simulink model "RealtimeModel"  (Simulink 7.0)
settings: Solver=FixedStepDiscrete  SolverMode=MultiTasking  StartTime=0.0  StopTime=RunningTime  FixedStep=sample  RelTol=1e-3
values from neighbouring files (symbols this model uses):
  Integrator = InitializeIntegrator(Integrator, Structure)    [RealtimeModel_Setup.m]
  SampleRate = Integrator.Timestep    [RealtimeModel_Setup.m]
  Structure = CalculateMatrices(Structure, Elements)    [RealtimeModel_Setup.m]
undefined symbols (not defined in the file or in its folder): Elements
libraries: simulink x2
(part 1 of 11)
settings Model: Creator=Tommy  LastModifiedBy=Tommy  BufferReuse=off
settings OptimizationCC: BlockReduction=off  OptimizeBlockIOStorage=off  BufferReuse=off  ExpressionFolding=off  LocalBlockOutputs=off
settings RTWCC: SystemTargetFile=xpctarget.tlc  TemplateMakefile=xpc_default_tmf  Description=xPC Target  ProcessScript=xpctarget_make_rtw_hook
settings xpcTargetCC: TargetFcnLib=ansi_tfl_table_tmw.mat  GenFloatMathFcnCalls=ANSI_C  CompOptLevelCompliant=off  PortableWordSizes=off
settings CustomProperty: DataType=string  Value=Real-Time

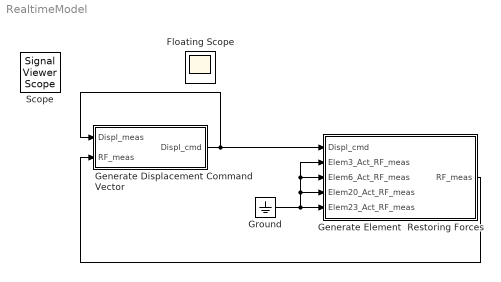
== system RealtimeModel ==
  Generate Displacement Command Vector : Subsystem
      mask Type: Generate Displacement Command Vector
      mask Description:
      | Generates the Displacement vector using the CR Algorithm.
      | 
      | Connect the measured displacement vector and measured restoring force vector to the inputs.
  Generate Element  Restoring Forces : Subsystem  TreatAsAtomicUnit=on  SystemSampleTime=SampleRate
  Ground : Ground
  Floating Scope : Scope
      settings: Floating=on
  Scope : SignalViewerScope  IOType=viewer  SampleTime=-1  RefreshTime=0.035000
  wires:
  Generate Displacement Command Vector/1(Displ_cmd) -> Generate Displacement Command Vector/1(Displ_meas), Generate Element  Restoring Forces/1(Displ_cmd)
  Generate Element  Restoring Forces/1(RF_meas) -> Generate Displacement Command Vector/2(RF_meas)
  Ground/1 -> Generate Element  Restoring Forces/5(Elem23_Act_RF_meas), Generate Element  Restoring Forces/4(Elem20_Act_RF_meas), Generate Element  Restoring Forces/3(Elem6_Act_RF_meas), Generate Element  Restoring Forces/2(Elem3_Act_RF_meas)

== system RealtimeModel/Generate Displacement Command Vector ==
  Displ_meas : Inport  OutDataType=sfix(16)  OutScaling=2^0
  RF_meas : Inport  Port=2  OutDataType=sfix(16)  OutScaling=2^0
  Constant : Constant  Value=Integrator.Alpha1  OutDataType=sfix(16)  OutScaling=2^0
  Constant1 : Constant  Value=Integrator.Alpha2  OutDataType=sfix(16)  OutScaling=2^0
  Constant2 : Constant  Value=Integrator.Timestep  OutDataType=sfix(16)  OutScaling=2^0
  Constant3 : Constant  Value=Integrator.PEFF  OutDataType=sfix(16)  OutScaling=2^0
  Data Store Acceleration : DataStoreMemory  DataStoreName=Acceleration  InitialValue=Integrator.Acceleration  OutDataType=sfix(16)  OutScaling=2^0
  Data Store DampingMatrixFree : DataStoreMemory  DataStoreName=DampingMatrixFree  InitialValue=Structure.DampingMatrixFree  OutDataType=sfix(16)  OutScaling=2^0
  Data Store Displacement : DataStoreMemory  DataStoreName=Displacement  InitialValue=Integrator.Displacement  OutDataType=sfix(16)  OutScaling=2^0
  Data Store MassMatrixFreeInv : DataStoreMemory  DataStoreName=MassMatrixFreeInv  InitialValue=Structure.MassMatrixFreeInv  OutDataType=sfix(16)  OutScaling=2^0
  Data Store Read Acceleration : DataStoreRead  DataStoreName=Acceleration  SampleTime=SampleRate
  Data Store Read DampingMatrixFree : DataStoreRead  DataStoreName=DampingMatrixFree  SampleTime=SampleRate
  Data Store Read Displacement : DataStoreRead  DataStoreName=Displacement  SampleTime=SampleRate
  Data Store Read MassMatrixFreeInv : DataStoreRead  DataStoreName=MassMatrixFreeInv  SampleTime=SampleRate
  Data Store Read Velocity : DataStoreRead  DataStoreName=Velocity  SampleTime=SampleRate
  Data Store Velocity : DataStoreMemory  DataStoreName=Velocity  InitialValue=Integrator.Velocity  OutDataType=sfix(16)  OutScaling=2^0
  Data Store Write Acceleration : DataStoreWrite  DataStoreName=Acceleration  SampleTime=-1
  Data Store Write Displacement : DataStoreWrite  DataStoreName=Displacement  SampleTime=-1
  Data Store Write Velocity : DataStoreWrite  DataStoreName=Velocity  SampleTime=-1
  Generate Acceleration Vector : Stateflow chart  TreatAsAtomicUnit=on  SystemSampleTime=SampleRate
  Generate Command Vectors : Stateflow chart  TreatAsAtomicUnit=on  SystemSampleTime=SampleRate
  Integration Step Count : Subsystem  TreatAsAtomicUnit=on  SystemSampleTime=SampleRate
      mask Type: Step count
      mask Description: Generates the step count
  Displ_cmd : Outport  OutDataType=sfix(16)  OutScaling=2^0
  wires:
  Generate Command Vectors/1(Displacement_v) -> Displ_cmd/1
  Constant2/1 -> Generate Command Vectors/1(Timestep)
  Constant1/1 -> Generate Command Vectors/3(Alpha2)
  Data Store Read Displacement/1 -> Generate Command Vectors/4(Displacement)
  Data Store Read Velocity/1 -> Generate Command Vectors/5(Velocity)
  Data Store Read Acceleration/1 -> Generate Command Vectors/6(Acceleration)
  Constant/1 -> Generate Command Vectors/2(Alpha1)
  Displ_meas/1 -> Data Store Write Displacement/1
  RF_meas/1 -> Generate Acceleration Vector/2(TotalRF)
  Generate Command Vectors/2(Velocity_v) -> Data Store Write Velocity/1, Generate Acceleration Vector/1(Velocity)
  Generate Acceleration Vector/1(Acceleration) -> Data Store Write Acceleration/1
  Constant3/1 -> Generate Acceleration Vector/3(PEFF)
  Data Store Read MassMatrixFreeInv/1 -> Generate Acceleration Vector/4(M_FreeInv)
  Data Store Read DampingMatrixFree/1 -> Generate Acceleration Vector/5(C_Free)
  Integration Step Count/1(Step Count) -> Generate Acceleration Vector/6(step_count)

== system RealtimeModel/Generate Element  Restoring Forces ==
  Displ_cmd : Inport  OutDataType=sfix(16)  OutScaling=2^0
  Elem3_Act_RF_meas : Inport  Port=2  OutDataType=sfix(16)  OutScaling=2^0
  Elem6_Act_RF_meas : Inport  Port=3  OutDataType=sfix(16)  OutScaling=2^0
  Elem20_Act_RF_meas : Inport  Port=4  OutDataType=sfix(16)  OutScaling=2^0
  Elem23_Act_RF_meas : Inport  Port=5  OutDataType=sfix(16)  OutScaling=2^0
  Form Total Restoring Force Vector : Subsystem  TreatAsAtomicUnit=on  SystemSampleTime=SampleRate
      mask Type: Form Restoring Force Vector
      mask Description:
      | Takes the restoring force vectors from each Element and combines them to form a total restoring force vector.
      | 
      | Connect the "Nodes_muxed" signal to the output of a Mux block which takes in all the Element "Nodes" outputs in order of ID.
      | 
      | Connect the "RF_muxed" signal to the output of a Mux block which takes in all the Element "RF" outputs in order of ID.
  Generate Type 1  Element Restoring Force Element 11 : Subsystem  TreatAsAtomicUnit=on  SystemSampleTime=SampleRate  mask(Generate Type 1 Element Restoring Force){id=11}
      mask prompts: id "Element ID"
      mask help:
      | Generates the Restoring Force vector for a Type 1 Element
      |
      | Enter the ID for this element corresponding with the input configuration file
  Generate Type 1  Element Restoring Force Element 12 : Subsystem  TreatAsAtomicUnit=on  SystemSampleTime=SampleRate  mask(Generate Type 1 Element Restoring Force){id=12}
      mask prompts: id "Element ID"
      mask help:
      | Generates the Restoring Force vector for a Type 1 Element
      |
      | Enter the ID for this element corresponding with the input configuration file
  Generate Type 1  Element Restoring Force Element 14 : Subsystem  TreatAsAtomicUnit=on  SystemSampleTime=SampleRate  mask(Generate Type 1 Element Restoring Force){id=14}
      mask prompts: id "Element ID"
      mask help:
      | Generates the Restoring Force vector for a Type 1 Element
      |
      | Enter the ID for this element corresponding with the input configuration file
  Generate Type 1  Element Restoring Force Element 15 : Subsystem  TreatAsAtomicUnit=on  SystemSampleTime=SampleRate  mask(Generate Type 1 Element Restoring Force){id=15}
      mask prompts: id "Element ID"
      mask help:
      | Generates the Restoring Force vector for a Type 1 Element
      |
      | Enter the ID for this element corresponding with the input configuration file
  Generate Type 1  Element Restoring Force Element 28 : Subsystem  TreatAsAtomicUnit=on  SystemSampleTime=SampleRate  mask(Generate Type 1 Element Restoring Force){id=28}
      mask prompts: id "Element ID"
      mask help:
      | Generates the Restoring Force vector for a Type 1 Element
      |
      | Enter the ID for this element corresponding with the input configuration file
  Generate Type 1  Element Restoring Force Element 29 : Subsystem  TreatAsAtomicUnit=on  SystemSampleTime=SampleRate  mask(Generate Type 1 Element Restoring Force){id=29}
      mask prompts: id "Element ID"
      mask help:
      | Generates the Restoring Force vector for a Type 1 Element
      |
      | Enter the ID for this element corresponding with the input configuration file
  Generate Type 1  Element Restoring Force Element 31 : Subsystem  TreatAsAtomicUnit=on  SystemSampleTime=SampleRate  mask(Generate Type 1 Element Restoring Force){id=31}
      mask prompts: id "Element ID"
      mask help:
      | Generates the Restoring Force vector for a Type 1 Element
      |
      | Enter the ID for this element corresponding with the input configuration file
  Generate Type 1  Element Restoring Force Element 32 : Subsystem  TreatAsAtomicUnit=on  SystemSampleTime=SampleRate  mask(Generate Type 1 Element Restoring Force){id=32}
      mask prompts: id "Element ID"
      mask help:
      | Generates the Restoring Force vector for a Type 1 Element
      |
      | Enter the ID for this element corresponding with the input configuration file
  Generate Type 2 Element Restoring Force Element 20 : Subsystem  TreatAsAtomicUnit=on  SystemSampleTime=SampleRate  mask(Generate Type 2 Element Restoring Force){id=20, simulation=off}
      mask prompts: id "Element ID"; simulation "Experiment Mode"
      mask help:
      | Generates the Restoring Force vector for a Type 2 Element
      |
      | Enter the ID for this element corresponding with the input configuration file
      |
      | Check the "Experiment Mode" box to activate the Act_RF_meas input.
      | Connect the Actuator Restoring Force feedback to the input.
  Generate Type 2 Element Restoring Force Element 23 : Subsystem  TreatAsAtomicUnit=on  SystemSampleTime=SampleRate  mask(Generate Type 2 Element Restoring Force){id=23, simulation=off}
      mask prompts: id "Element ID"; simulation "Experiment Mode"
      mask help:
      | Generates the Restoring Force vector for a Type 2 Element
      |
      | Enter the ID for this element corresponding with the input configuration file
      |
      | Check the "Experiment Mode" box to activate the Act_RF_meas input.
      | Connect the Actuator Restoring Force feedback to the input.
  Generate Type 2 Element Restoring Force Element 3 : Subsystem  TreatAsAtomicUnit=on  SystemSampleTime=SampleRate  mask(Generate Type 2 Element Restoring Force){id=3, simulation=off}
      mask prompts: id "Element ID"; simulation "Experiment Mode"
      mask help:
      | Generates the Restoring Force vector for a Type 2 Element
      |
      | Enter the ID for this element corresponding with the input configuration file
      |
      | Check the "Experiment Mode" box to activate the Act_RF_meas input.
      | Connect the Actuator Restoring Force feedback to the input.
  Generate Type 2 Element Restoring Force Element 6 : Subsystem  TreatAsAtomicUnit=on  SystemSampleTime=SampleRate  mask(Generate Type 2 Element Restoring Force){id=6, simulation=off}
      mask prompts: id "Element ID"; simulation "Experiment Mode"
      mask help:
      | Generates the Restoring Force vector for a Type 2 Element
      |
      | Enter the ID for this element corresponding with the input configuration file
      |
      | Check the "Experiment Mode" box to activate the Act_RF_meas input.
      | Connect the Actuator Restoring Force feedback to the input.
  Generate Type 3  Element Restoring Force Element 1 : Subsystem  TreatAsAtomicUnit=on  SystemSampleTime=SampleRate  mask(Generate Type 3 Element Restoring Force){id=1}
      mask prompts: id "Element ID"
      mask help:
      | Generates the Restoring Force vector for a Type 3 Element
      |
      | Enter the ID for this element corresponding with the input configuration file
  Generate Type 3  Element Restoring Force Element 10 : Subsystem  TreatAsAtomicUnit=on  SystemSampleTime=SampleRate  mask(Generate Type 3 Element Restoring Force){id=10}
      mask prompts: id "Element ID"
      mask help:
      | Generates the Restoring Force vector for a Type 3 Element
      |
      | Enter the ID for this element corresponding with the input configuration file
  Generate Type 3  Element Restoring Force Element 13 : Subsystem  TreatAsAtomicUnit=on  SystemSampleTime=SampleRate  mask(Generate Type 3 Element Restoring Force){id=13}
      mask prompts: id "Element ID"
      mask help:
      | Generates the Restoring Force vector for a Type 3 Element
      |
      | Enter the ID for this element corresponding with the input configuration file
  Generate Type 3  Element Restoring Force Element 16 : Subsystem  TreatAsAtomicUnit=on  SystemSampleTime=SampleRate  mask(Generate Type 3 Element Restoring Force){id=16}
      mask prompts: id "Element ID"
      mask help:
      | Generates the Restoring Force vector for a Type 3 Element
      |
      | Enter the ID for this element corresponding with the input configuration file
  Generate Type 3  Element Restoring Force Element 17 : Subsystem  TreatAsAtomicUnit=on  SystemSampleTime=SampleRate  mask(Generate Type 3 Element Restoring Force){id=17}
      mask prompts: id "Element ID"
      mask help:
      | Generates the Restoring Force vector for a Type 3 Element
      |
      | Enter the ID for this element corresponding with the input configuration file
  Generate Type 3  Element Restoring Force Element 18 : Subsystem  TreatAsAtomicUnit=on  SystemSampleTime=SampleRate  mask(Generate Type 3 Element Restoring Force){id=18}
      mask prompts: id "Element ID"
      mask help:
      | Generates the Restoring Force vector for a Type 3 Element
      |
      | Enter the ID for this element corresponding with the input configuration file
  Generate Type 3  Element Restoring Force Element 19 : Subsystem  TreatAsAtomicUnit=on  SystemSampleTime=SampleRate  mask(Generate Type 3 Element Restoring Force){id=19}
      mask prompts: id "Element ID"
      mask help:
      | Generates the Restoring Force vector for a Type 3 Element
      |
      | Enter the ID for this element corresponding with the input configuration file
  Generate Type 3  Element Restoring Force Element 2 : Subsystem  TreatAsAtomicUnit=on  SystemSampleTime=SampleRate  mask(Generate Type 3 Element Restoring Force){id=2}
      mask prompts: id "Element ID"
      mask help:
      | Generates the Restoring Force vector for a Type 3 Element
      |
      | Enter the ID for this element corresponding with the input configuration file
  Generate Type 3  Element Restoring Force Element 21 : Subsystem  TreatAsAtomicUnit=on  SystemSampleTime=SampleRate  mask(Generate Type 3 Element Restoring Force){id=21}
      mask prompts: id "Element ID"
      mask help:
      | Generates the Restoring Force vector for a Type 3 Element
      |
      | Enter the ID for this element corresponding with the input configuration file
  Generate Type 3  Element Restoring Force Element 22 : Subsystem  TreatAsAtomicUnit=on  SystemSampleTime=SampleRate  mask(Generate Type 3 Element Restoring Force){id=22}
      mask prompts: id "Element ID"
      mask help:
      | Generates the Restoring Force vector for a Type 3 Element
      |
      | Enter the ID for this element corresponding with the input configuration file
  Generate Type 3  Element Restoring Force Element 24 : Subsystem  TreatAsAtomicUnit=on  SystemSampleTime=SampleRate  mask(Generate Type 3 Element Restoring Force){id=24}
      mask prompts: id "Element ID"
      mask help:
      | Generates the Restoring Force vector for a Type 3 Element
      |
      | Enter the ID for this element corresponding with the input configuration file
  Generate Type 3  Element Restoring Force Element 25 : Subsystem  TreatAsAtomicUnit=on  SystemSampleTime=SampleRate  mask(Generate Type 3 Element Restoring Force){id=25}
      mask prompts: id "Element ID"
      mask help:
      | Generates the Restoring Force vector for a Type 3 Element
      |
      | Enter the ID for this element corresponding with the input configuration file
  Generate Type 3  Element Restoring Force Element 26 : Subsystem  TreatAsAtomicUnit=on  SystemSampleTime=SampleRate  mask(Generate Type 3 Element Restoring Force){id=26}
      mask prompts: id "Element ID"
      mask help:
      | Generates the Restoring Force vector for a Type 3 Element
      |
      | Enter the ID for this element corresponding with the input configuration file
  Generate Type 3  Element Restoring Force Element 27 : Subsystem  TreatAsAtomicUnit=on  SystemSampleTime=SampleRate  mask(Generate Type 3 Element Restoring Force){id=27}
      mask prompts: id "Element ID"
      mask help:
      | Generates the Restoring Force vector for a Type 3 Element
      |
      | Enter the ID for this element corresponding with the input configuration file
  Generate Type 3  Element Restoring Force Element 30 : Subsystem  TreatAsAtomicUnit=on  SystemSampleTime=SampleRate  mask(Generate Type 3 Element Restoring Force){id=30}
      mask prompts: id "Element ID"
      mask help:
      | Generates the Restoring Force vector for a Type 3 Element
      |
      | Enter the ID for this element corresponding with the input configuration file
  Generate Type 3  Element Restoring Force Element 33 : Subsystem  TreatAsAtomicUnit=on  SystemSampleTime=SampleRate  mask(Generate Type 3 Element Restoring Force){id=33}
      mask prompts: id "Element ID"
      mask help:
      | Generates the Restoring Force vector for a Type 3 Element
      |
      | Enter the ID for this element corresponding with the input configuration file
  Generate Type 3  Element Restoring Force Element 34 : Subsystem  TreatAsAtomicUnit=on  SystemSampleTime=SampleRate  mask(Generate Type 3 Element Restoring Force){id=34}
      mask prompts: id "Element ID"
      mask help:
      | Generates the Restoring Force vector for a Type 3 Element
      |
      | Enter the ID for this element corresponding with the input configuration file
  Generate Type 3  Element Restoring Force Element 4 : Subsystem  TreatAsAtomicUnit=on  SystemSampleTime=SampleRate  mask(Generate Type 3 Element Restoring Force){id=4}
      mask prompts: id "Element ID"
      mask help:
      | Generates the Restoring Force vector for a Type 3 Element
      |
      | Enter the ID for this element corresponding with the input configuration file
  Generate Type 3  Element Restoring Force Element 5 : Subsystem  TreatAsAtomicUnit=on  SystemSampleTime=SampleRate  mask(Generate Type 3 Element Restoring Force){id=5}
      mask prompts: id "Element ID"
      mask help:
      | Generates the Restoring Force vector for a Type 3 Element
      |
      | Enter the ID for this element corresponding with the input configuration file
  Generate Type 3  Element Restoring Force Element 7 : Subsystem  TreatAsAtomicUnit=on  SystemSampleTime=SampleRate  mask(Generate Type 3 Element Restoring Force){id=7}
      mask prompts: id "Element ID"
      mask help:
      | Generates the Restoring Force vector for a Type 3 Element
      |
      | Enter the ID for this element corresponding with the input configuration file
  Generate Type 3  Element Restoring Force Element 8 : Subsystem  TreatAsAtomicUnit=on  SystemSampleTime=SampleRate  mask(Generate Type 3 Element Restoring Force){id=8}
      mask prompts: id "Element ID"
      mask help:
      | Generates the Restoring Force vector for a Type 3 Element
      |
      | Enter the ID for this element corresponding with the input configuration file
  Generate Type 3  Element Restoring Force Element 9 : Subsystem  TreatAsAtomicUnit=on  SystemSampleTime=SampleRate  mask(Generate Type 3 Element Restoring Force){id=9}
      mask prompts: id "Element ID"
      mask help:
      | Generates the Restoring Force vector for a Type 3 Element
      |
      | Enter the ID for this element corresponding with the input configuration file
  "Generate Type 4  Element Restoring Force Element 35 " : Subsystem  TreatAsAtomicUnit=on  SystemSampleTime=SampleRate  mask(Generate Type 4 Element Restoring Force){id=35}
      mask prompts: id "Element ID"
      mask help:
      | Generates the Restoring Force vector for a Type 4 Element
      |
      | Enter the ID for this element corresponding with the input configuration file
  Nodes_Mux : Mux  Inputs=35
  RF_Mux : Mux  Inputs=35
  RF_meas : Outport  OutDataType=sfix(16)  OutScaling=2^0
  wires:
  Form Total Restoring Force Vector/1(Total RF) -> RF_meas/1
  Nodes_Mux/1 -> Form Total Restoring Force Vector/1(Nodes_Muxed)
  RF_Mux/1 -> Form Total Restoring Force Vector/2(RF_muxed)
  Elem3_Act_RF_meas/1 -> Generate Type 2 Element Restoring Force Element 3/2(Act_RF_meas)
  Elem6_Act_RF_meas/1 -> Generate Type 2 Element Restoring Force Element 6/2(Act_RF_meas)
  Elem20_Act_RF_meas/1 -> Generate Type 2 Element Restoring Force Element 20/2(Act_RF_meas)
  Elem23_Act_RF_meas/1 -> Generate Type 2 Element Restoring Force Element 23/2(Act_RF_meas)
  Displ_cmd/1 -> Generate Type 3  Element Restoring Force Element 1/1(Displ_cmd), Generate Type 3  Element Restoring Force Element 2/1(Displ_cmd), Generate Type 2 Element Restoring Force Element 3/1(Displ_cmd), Generate Type 3  Element Restoring Force Element 4/1(Displ_cmd), Generate Type 3  Element Restoring Force Element 5/1(Displ_cmd), Generate Type 2 Element Restoring Force Element 6/1(Displ_cmd), Generate Type 3  Element Restoring Force Element 7/1(Displ_cmd), Generate Type 3  Element Restoring Force Element 8/1(Displ_cmd), Generate Type 3  Element Restoring Force Element 9/1(Displ_cmd), Generate Type 3  Element Restoring Force Element 10/1(Displ_cmd), Generate Type 1  Element Restoring Force Element 11/1(Displ_cmd), Generate Type 1  Element Restoring Force Element 12/1(Displ_cmd), Generate Type 3  Element Restoring Force Element 13/1(Displ_cmd), Generate Type 1  Element Restoring Force Element 14/1(Displ_cmd), Generate Type 1  Element Restoring Force Element 15/1(Displ_cmd), Generate Type 3  Element Restoring Force Element 16/1(Displ_cmd), Generate Type 3  Element Restoring Force Element 17/1(Displ_cmd), Generate Type 3  Element Restoring Force Element 18/1(Displ_cmd), Generate Type 3  Element Restoring Force Element 19/1(Displ_cmd), Generate Type 2 Element Restoring Force Element 20/1(Displ_cmd), Generate Type 3  Element Restoring Force Element 21/1(Displ_cmd), Generate Type 3  Element Restoring Force Element 22/1(Displ_cmd), Generate Type 2 Element Restoring Force Element 23/1(Displ_cmd), Generate Type 3  Element Restoring Force Element 24/1(Displ_cmd), Generate Type 3  Element Restoring Force Element 25/1(Displ_cmd), Generate Type 3  Element Restoring Force Element 26/1(Displ_cmd), Generate Type 3  Element Restoring Force Element 27/1(Displ_cmd), Generate Type 1  Element Restoring Force Element 28/1(Displ_cmd), Generate Type 1  Element Restoring Force Element 29/1(Displ_cmd), Generate Type 3  Element Restoring Force Element 30/1(Displ_cmd), Generate Type 1  Element Restoring Force Element 31/1(Displ_cmd), Generate Type 1  Element Restoring Force Element 32/1(Displ_cmd), Generate Type 3  Element Restoring Force Element 33/1(Displ_cmd), Generate Type 3  Element Restoring Force Element 34/1(Displ_cmd), "Generate Type 4  Element Restoring Force Element 35 "/1(Displ_cmd)
  Generate Type 3  Element Restoring Force Element 1/1(Nodes) -> Nodes_Mux/1
  Generate Type 3  Element Restoring Force Element 2/1(Nodes) -> Nodes_Mux/2
  Generate Type 2 Element Restoring Force Element 3/1(Nodes) -> Nodes_Mux/3
  Generate Type 3  Element Restoring Force Element 4/1(Nodes) -> Nodes_Mux/4
  Generate Type 3  Element Restoring Force Element 5/1(Nodes) -> Nodes_Mux/5
  Generate Type 2 Element Restoring Force Element 6/1(Nodes) -> Nodes_Mux/6
  Generate Type 3  Element Restoring Force Element 7/1(Nodes) -> Nodes_Mux/7
  Generate Type 3  Element Restoring Force Element 8/1(Nodes) -> Nodes_Mux/8
  Generate Type 3  Element Restoring Force Element 9/1(Nodes) -> Nodes_Mux/9
  Generate Type 3  Element Restoring Force Element 10/1(Nodes) -> Nodes_Mux/10
  Generate Type 1  Element Restoring Force Element 11/1(Nodes) -> Nodes_Mux/11
  Generate Type 1  Element Restoring Force Element 12/1(Nodes) -> Nodes_Mux/12
  Generate Type 3  Element Restoring Force Element 13/1(Nodes) -> Nodes_Mux/13
  Generate Type 1  Element Restoring Force Element 14/1(Nodes) -> Nodes_Mux/14
  Generate Type 1  Element Restoring Force Element 15/1(Nodes) -> Nodes_Mux/15
  Generate Type 3  Element Restoring Force Element 16/1(Nodes) -> Nodes_Mux/16
  Generate Type 3  Element Restoring Force Element 17/1(Nodes) -> Nodes_Mux/17
  Generate Type 3  Element Restoring Force Element 18/1(Nodes) -> Nodes_Mux/18
  Generate Type 3  Element Restoring Force Element 19/1(Nodes) -> Nodes_Mux/19
  Generate Type 2 Element Restoring Force Element 20/1(Nodes) -> Nodes_Mux/20
  Generate Type 3  Element Restoring Force Element 21/1(Nodes) -> Nodes_Mux/21
  Generate Type 3  Element Restoring Force Element 22/1(Nodes) -> Nodes_Mux/22
  Generate Type 2 Element Restoring Force Element 23/1(Nodes) -> Nodes_Mux/23
  Generate Type 3  Element Restoring Force Element 24/1(Nodes) -> Nodes_Mux/24
  Generate Type 3  Element Restoring Force Element 25/1(Nodes) -> Nodes_Mux/25
  Generate Type 3  Element Restoring Force Element 26/1(Nodes) -> Nodes_Mux/26
  Generate Type 3  Element Restoring Force Element 27/1(Nodes) -> Nodes_Mux/27
  Generate Type 1  Element Restoring Force Element 28/1(Nodes) -> Nodes_Mux/28
  Generate Type 1  Element Restoring Force Element 29/1(Nodes) -> Nodes_Mux/29
  Generate Type 3  Element Restoring Force Element 30/1(Nodes) -> Nodes_Mux/30
  Generate Type 1  Element Restoring Force Element 31/1(Nodes) -> Nodes_Mux/31
  Generate Type 3  Element Restoring Force Element 34/1(Nodes) -> Nodes_Mux/34
  "Generate Type 4  Element Restoring Force Element 35 "/1(Nodes) -> Nodes_Mux/35
  Generate Type 1  Element Restoring Force Element 32/1(Nodes) -> Nodes_Mux/32
  Generate Type 3  Element Restoring Force Element 33/1(Nodes) -> Nodes_Mux/33
  "Generate Type 4  Element Restoring Force Element 35 "/2(RF) -> RF_Mux/35
  Generate Type 3  Element Restoring Force Element 34/2(RF) -> RF_Mux/34
  Generate Type 3  Element Restoring Force Element 33/2(RF) -> RF_Mux/33
  Generate Type 1  Element Restoring Force Element 32/2(RF) -> RF_Mux/32
  Generate Type 1  Element Restoring Force Element 31/2(RF) -> RF_Mux/31
  Generate Type 3  Element Restoring Force Element 30/2(RF) -> RF_Mux/30
  Generate Type 1  Element Restoring Force Element 29/2(RF) -> RF_Mux/29
  Generate Type 1  Element Restoring Force Element 28/2(RF) -> RF_Mux/28
  Generate Type 3  Element Restoring Force Element 27/2(RF) -> RF_Mux/27
  Generate Type 3  Element Restoring Force Element 26/2(RF) -> RF_Mux/26
  Generate Type 3  Element Restoring Force Element 25/2(RF) -> RF_Mux/25
  Generate Type 3  Element Restoring Force Element 24/2(RF) -> RF_Mux/24
  Generate Type 2 Element Restoring Force Element 23/2(RF) -> RF_Mux/23
  Generate Type 3  Element Restoring Force Element 22/2(RF) -> RF_Mux/22
  Generate Type 3  Element Restoring Force Element 21/2(RF) -> RF_Mux/21
  Generate Type 2 Element Restoring Force Element 20/2(RF) -> RF_Mux/20
  Generate Type 3  Element Restoring Force Element 19/2(RF) -> RF_Mux/19
  Generate Type 3  Element Restoring Force Element 18/2(RF) -> RF_Mux/18
  Generate Type 3  Element Restoring Force Element 17/2(RF) -> RF_Mux/17
  Generate Type 3  Element Restoring Force Element 16/2(RF) -> RF_Mux/16
  Generate Type 1  Element Restoring Force Element 15/2(RF) -> RF_Mux/15
  Generate Type 1  Element Restoring Force Element 14/2(RF) -> RF_Mux/14
  Generate Type 3  Element Restoring Force Element 13/2(RF) -> RF_Mux/13
  Generate Type 1  Element Restoring Force Element 12/2(RF) -> RF_Mux/12
  Generate Type 1  Element Restoring Force Element 11/2(RF) -> RF_Mux/11
  Generate Type 3  Element Restoring Force Element 10/2(RF) -> RF_Mux/10
  Generate Type 3  Element Restoring Force Element 9/2(RF) -> RF_Mux/9
  Generate Type 3  Element Restoring Force Element 8/2(RF) -> RF_Mux/8
  Generate Type 3  Element Restoring Force Element 7/2(RF) -> RF_Mux/7
  Generate Type 2 Element Restoring Force Element 6/2(RF) -> RF_Mux/6
  Generate Type 3  Element Restoring Force Element 5/2(RF) -> RF_Mux/5
  Generate Type 3  Element Restoring Force Element 4/2(RF) -> RF_Mux/4
  Generate Type 2 Element Restoring Force Element 3/2(RF) -> RF_Mux/3
  Generate Type 3  Element Restoring Force Element 2/2(RF) -> RF_Mux/2
  Generate Type 3  Element Restoring Force Element 1/2(RF) -> RF_Mux/1

== system RealtimeModel/Generate Displacement Command Vector/Integration Step Count ==
  Increment Stored Integer : simulink/Additional Math & Discrete/Additional Math: Increment - Decrement/Increment Stored Integer  SystemSampleTime=-1
  step count : simulink/Sources/Counter Free-Running  SystemSampleTime=-1  NumBits=32  tsamp=-1
  Step Count : Outport  OutDataType=sfix(16)  OutScaling=2^0
  wires:
  step count/1 -> Increment Stored Integer/1
  Increment Stored Integer/1 -> Step Count/1

== system RealtimeModel/Generate Element  Restoring Forces/Form Total Restoring Force Vector ==
  Nodes_Muxed : Inport  OutDataType=sfix(16)  OutScaling=2^0
  RF_muxed : Inport  Port=2  OutDataType=sfix(16)  OutScaling=2^0
  Form Restoring Force Vector : Stateflow chart  TreatAsAtomicUnit=on  SystemSampleTime=SampleRate
  Total RF : Outport  OutDataType=sfix(16)  OutScaling=2^0
  wires:
  RF_muxed/1 -> Form Restoring Force Vector/2(RF_muxed)
  Form Restoring Force Vector/1(TotalRF) -> Total RF/1
  Nodes_Muxed/1 -> Form Restoring Force Vector/1(Nodes_muxed)

== system RealtimeModel/Generate Element  Restoring Forces/Generate Type 1  Element Restoring Force Element 11 ==
  Displ_cmd : Inport  OutDataType=sfix(16)  OutScaling=2^0
  Constant : Constant  Value=Structure.NumFreeDOF  OutDataType=sfix(16)  OutScaling=2^0
  "Type 1 Element " : Subsystem  mask(Element Type 1){id=id}
      mask prompts: id "Element ID:"
      mask help: Enter the ID for this element corresponding with the input configuration file
  Type 1 Element RF : Stateflow chart  TreatAsAtomicUnit=on  SystemSampleTime=SampleRate
  Nodes : Outport  OutDataType=sfix(16)  OutScaling=2^0
  RF : Outport  Port=2  OutDataType=sfix(16)  OutScaling=2^0
  wires:
  Constant/1 -> Type 1 Element RF/2(NumFreeDOF)
  Type 1 Element RF/1(Nodes) -> Nodes/1
  Type 1 Element RF/2(RF) -> RF/1
  Displ_cmd/1 -> Type 1 Element RF/3(Displacement)
  "Type 1 Element "/1(Element) -> Type 1 Element RF/1(Element)

== system RealtimeModel/Generate Element  Restoring Forces/Generate Type 1  Element Restoring Force Element 12 ==
  Displ_cmd : Inport  OutDataType=sfix(16)  OutScaling=2^0
  Constant : Constant  Value=Structure.NumFreeDOF  OutDataType=sfix(16)  OutScaling=2^0
  "Type 1 Element " : Subsystem  mask(Element Type 1){id=id}
      mask prompts: id "Element ID:"
      mask help: Enter the ID for this element corresponding with the input configuration file
  Type 1 Element RF : Stateflow chart  TreatAsAtomicUnit=on  SystemSampleTime=SampleRate
  Nodes : Outport  OutDataType=sfix(16)  OutScaling=2^0
  RF : Outport  Port=2  OutDataType=sfix(16)  OutScaling=2^0
  wires:
  "Type 1 Element "/1(Element) -> Type 1 Element RF/1(Element)
  Displ_cmd/1 -> Type 1 Element RF/3(Displacement)
  Type 1 Element RF/2(RF) -> RF/1
  Type 1 Element RF/1(Nodes) -> Nodes/1
  Constant/1 -> Type 1 Element RF/2(NumFreeDOF)

== system RealtimeModel/Generate Element  Restoring Forces/Generate Type 1  Element Restoring Force Element 14 ==
  Displ_cmd : Inport  OutDataType=sfix(16)  OutScaling=2^0
  Constant : Constant  Value=Structure.NumFreeDOF  OutDataType=sfix(16)  OutScaling=2^0
  "Type 1 Element " : Subsystem  mask(Element Type 1){id=id}
      mask prompts: id "Element ID:"
      mask help: Enter the ID for this element corresponding with the input configuration file
  Type 1 Element RF : Stateflow chart  TreatAsAtomicUnit=on  SystemSampleTime=SampleRate
  Nodes : Outport  OutDataType=sfix(16)  OutScaling=2^0
  RF : Outport  Port=2  OutDataType=sfix(16)  OutScaling=2^0
  wires:
  Constant/1 -> Type 1 Element RF/2(NumFreeDOF)
  Type 1 Element RF/1(Nodes) -> Nodes/1
  Type 1 Element RF/2(RF) -> RF/1
  Displ_cmd/1 -> Type 1 Element RF/3(Displacement)
  "Type 1 Element "/1(Element) -> Type 1 Element RF/1(Element)

== system RealtimeModel/Generate Element  Restoring Forces/Generate Type 1  Element Restoring Force Element 15 ==
  Displ_cmd : Inport  OutDataType=sfix(16)  OutScaling=2^0
  Constant : Constant  Value=Structure.NumFreeDOF  OutDataType=sfix(16)  OutScaling=2^0
  "Type 1 Element " : Subsystem  mask(Element Type 1){id=id}
      mask prompts: id "Element ID:"
      mask help: Enter the ID for this element corresponding with the input configuration file
  Type 1 Element RF : Stateflow chart  TreatAsAtomicUnit=on  SystemSampleTime=SampleRate
  Nodes : Outport  OutDataType=sfix(16)  OutScaling=2^0
  RF : Outport  Port=2  OutDataType=sfix(16)  OutScaling=2^0
  wires:
  "Type 1 Element "/1(Element) -> Type 1 Element RF/1(Element)
  Displ_cmd/1 -> Type 1 Element RF/3(Displacement)
  Type 1 Element RF/2(RF) -> RF/1
  Type 1 Element RF/1(Nodes) -> Nodes/1
  Constant/1 -> Type 1 Element RF/2(NumFreeDOF)

== system RealtimeModel/Generate Element  Restoring Forces/Generate Type 1  Element Restoring Force Element 28 ==
  Displ_cmd : Inport  OutDataType=sfix(16)  OutScaling=2^0
  Constant : Constant  Value=Structure.NumFreeDOF  OutDataType=sfix(16)  OutScaling=2^0
  "Type 1 Element " : Subsystem  mask(Element Type 1){id=id}
      mask prompts: id "Element ID:"
      mask help: Enter the ID for this element corresponding with the input configuration file
  Type 1 Element RF : Stateflow chart  TreatAsAtomicUnit=on  SystemSampleTime=SampleRate
  Nodes : Outport  OutDataType=sfix(16)  OutScaling=2^0
  RF : Outport  Port=2  OutDataType=sfix(16)  OutScaling=2^0
  wires:
  Constant/1 -> Type 1 Element RF/2(NumFreeDOF)
  Type 1 Element RF/1(Nodes) -> Nodes/1
  Type 1 Element RF/2(RF) -> RF/1
  Displ_cmd/1 -> Type 1 Element RF/3(Displacement)
  "Type 1 Element "/1(Element) -> Type 1 Element RF/1(Element)

== system RealtimeModel/Generate Element  Restoring Forces/Generate Type 1  Element Restoring Force Element 29 ==
  Displ_cmd : Inport  OutDataType=sfix(16)  OutScaling=2^0
  Constant : Constant  Value=Structure.NumFreeDOF  OutDataType=sfix(16)  OutScaling=2^0
  "Type 1 Element " : Subsystem  mask(Element Type 1){id=id}
      mask prompts: id "Element ID:"
      mask help: Enter the ID for this element corresponding with the input configuration file
  Type 1 Element RF : Stateflow chart  TreatAsAtomicUnit=on  SystemSampleTime=SampleRate
  Nodes : Outport  OutDataType=sfix(16)  OutScaling=2^0
  RF : Outport  Port=2  OutDataType=sfix(16)  OutScaling=2^0
  wires:
  "Type 1 Element "/1(Element) -> Type 1 Element RF/1(Element)
  Displ_cmd/1 -> Type 1 Element RF/3(Displacement)
  Type 1 Element RF/2(RF) -> RF/1
  Type 1 Element RF/1(Nodes) -> Nodes/1
  Constant/1 -> Type 1 Element RF/2(NumFreeDOF)

== system RealtimeModel/Generate Element  Restoring Forces/Generate Type 1  Element Restoring Force Element 31 ==
  Displ_cmd : Inport  OutDataType=sfix(16)  OutScaling=2^0
  Constant : Constant  Value=Structure.NumFreeDOF  OutDataType=sfix(16)  OutScaling=2^0
  "Type 1 Element " : Subsystem  mask(Element Type 1){id=id}
      mask prompts: id "Element ID:"
      mask help: Enter the ID for this element corresponding with the input configuration file
  Type 1 Element RF : Stateflow chart  TreatAsAtomicUnit=on  SystemSampleTime=SampleRate
  Nodes : Outport  OutDataType=sfix(16)  OutScaling=2^0
  RF : Outport  Port=2  OutDataType=sfix(16)  OutScaling=2^0
  wires:
  Constant/1 -> Type 1 Element RF/2(NumFreeDOF)
  Type 1 Element RF/1(Nodes) -> Nodes/1
  Type 1 Element RF/2(RF) -> RF/1
  Displ_cmd/1 -> Type 1 Element RF/3(Displacement)
  "Type 1 Element "/1(Element) -> Type 1 Element RF/1(Element)

== system RealtimeModel/Generate Element  Restoring Forces/Generate Type 1  Element Restoring Force Element 32 ==
  Displ_cmd : Inport  OutDataType=sfix(16)  OutScaling=2^0
  Constant : Constant  Value=Structure.NumFreeDOF  OutDataType=sfix(16)  OutScaling=2^0
  "Type 1 Element " : Subsystem  mask(Element Type 1){id=id}
      mask prompts: id "Element ID:"
      mask help: Enter the ID for this element corresponding with the input configuration file
  Type 1 Element RF : Stateflow chart  TreatAsAtomicUnit=on  SystemSampleTime=SampleRate
  Nodes : Outport  OutDataType=sfix(16)  OutScaling=2^0
  RF : Outport  Port=2  OutDataType=sfix(16)  OutScaling=2^0
  wires:
  "Type 1 Element "/1(Element) -> Type 1 Element RF/1(Element)
  Displ_cmd/1 -> Type 1 Element RF/3(Displacement)
  Type 1 Element RF/2(RF) -> RF/1
  Type 1 Element RF/1(Nodes) -> Nodes/1
  Constant/1 -> Type 1 Element RF/2(NumFreeDOF)

== system RealtimeModel/Generate Element  Restoring Forces/Generate Type 2 Element Restoring Force Element 20 ==
  Displ_cmd : Inport  OutDataType=sfix(16)  OutScaling=2^0
  Act_RF_meas : Inport  Port=2  OutDataType=sfix(16)  OutScaling=2^0
  Constant : Constant  Value=Structure.NumFreeDOF  OutDataType=sfix(16)  OutScaling=2^0
  Constant1 : Constant  Value=simulation  OutDataType=sfix(16)  OutScaling=2^0
  Type 2 Element : Subsystem  mask(Element Type 2){id=id}
      mask prompts: id "Element ID:"
      mask help: Enter the ID for this element corresponding with the input configuration file
  Type 2 Element RF : Stateflow chart  TreatAsAtomicUnit=on  SystemSampleTime=SampleRate
  Nodes : Outport  OutDataType=sfix(16)  OutScaling=2^0
  RF : Outport  Port=2  OutDataType=sfix(16)  OutScaling=2^0
  wires:
  Type 2 Element/1(Element) -> Type 2 Element RF/1(Element)
  Act_RF_meas/1 -> Type 2 Element RF/4(ActuatorRF)
  Type 2 Element RF/1(Nodes) -> Nodes/1
  Type 2 Element RF/2(RF) -> RF/1
  Displ_cmd/1 -> Type 2 Element RF/3(Displacement)
  Constant/1 -> Type 2 Element RF/2(NumFreeDOF)
  Constant1/1 -> Type 2 Element RF/5(simulation)

== system RealtimeModel/Generate Element  Restoring Forces/Generate Type 2 Element Restoring Force Element 23 ==
  Displ_cmd : Inport  OutDataType=sfix(16)  OutScaling=2^0
  Act_RF_meas : Inport  Port=2  OutDataType=sfix(16)  OutScaling=2^0
  Constant : Constant  Value=Structure.NumFreeDOF  OutDataType=sfix(16)  OutScaling=2^0
  Constant1 : Constant  Value=simulation  OutDataType=sfix(16)  OutScaling=2^0
  Type 2 Element : Subsystem  mask(Element Type 2){id=id}
      mask prompts: id "Element ID:"
      mask help: Enter the ID for this element corresponding with the input configuration file
  Type 2 Element RF : Stateflow chart  TreatAsAtomicUnit=on  SystemSampleTime=SampleRate
  Nodes : Outport  OutDataType=sfix(16)  OutScaling=2^0
  RF : Outport  Port=2  OutDataType=sfix(16)  OutScaling=2^0
  wires:
  Type 2 Element/1(Element) -> Type 2 Element RF/1(Element)
  Act_RF_meas/1 -> Type 2 Element RF/4(ActuatorRF)
  Type 2 Element RF/1(Nodes) -> Nodes/1
  Type 2 Element RF/2(RF) -> RF/1
  Displ_cmd/1 -> Type 2 Element RF/3(Displacement)
  Constant/1 -> Type 2 Element RF/2(NumFreeDOF)
  Constant1/1 -> Type 2 Element RF/5(simulation)

== system RealtimeModel/Generate Element  Restoring Forces/Generate Type 2 Element Restoring Force Element 3 ==
  Displ_cmd : Inport  OutDataType=sfix(16)  OutScaling=2^0
  Act_RF_meas : Inport  Port=2  OutDataType=sfix(16)  OutScaling=2^0
  Constant : Constant  Value=Structure.NumFreeDOF  OutDataType=sfix(16)  OutScaling=2^0
  Constant1 : Constant  Value=simulation  OutDataType=sfix(16)  OutScaling=2^0
  Type 2 Element : Subsystem  mask(Element Type 2){id=id}
      mask prompts: id "Element ID:"
      mask help: Enter the ID for this element corresponding with the input configuration file
  Type 2 Element RF : Stateflow chart  TreatAsAtomicUnit=on  SystemSampleTime=SampleRate
  Nodes : Outport  OutDataType=sfix(16)  OutScaling=2^0
  RF : Outport  Port=2  OutDataType=sfix(16)  OutScaling=2^0
  wires:
  Type 2 Element/1(Element) -> Type 2 Element RF/1(Element)
  Act_RF_meas/1 -> Type 2 Element RF/4(ActuatorRF)
  Type 2 Element RF/1(Nodes) -> Nodes/1
  Type 2 Element RF/2(RF) -> RF/1
  Displ_cmd/1 -> Type 2 Element RF/3(Displacement)
  Constant/1 -> Type 2 Element RF/2(NumFreeDOF)
  Constant1/1 -> Type 2 Element RF/5(simulation)

== system RealtimeModel/Generate Element  Restoring Forces/Generate Type 2 Element Restoring Force Element 6 ==
  Displ_cmd : Inport  OutDataType=sfix(16)  OutScaling=2^0
  Act_RF_meas : Inport  Port=2  OutDataType=sfix(16)  OutScaling=2^0
  Constant : Constant  Value=Structure.NumFreeDOF  OutDataType=sfix(16)  OutScaling=2^0
  Constant1 : Constant  Value=simulation  OutDataType=sfix(16)  OutScaling=2^0
  Type 2 Element : Subsystem  mask(Element Type 2){id=id}
      mask prompts: id "Element ID:"
      mask help: Enter the ID for this element corresponding with the input configuration file
  Type 2 Element RF : Stateflow chart  TreatAsAtomicUnit=on  SystemSampleTime=SampleRate
  Nodes : Outport  OutDataType=sfix(16)  OutScaling=2^0
  RF : Outport  Port=2  OutDataType=sfix(16)  OutScaling=2^0
  wires:
  Type 2 Element/1(Element) -> Type 2 Element RF/1(Element)
  Act_RF_meas/1 -> Type 2 Element RF/4(ActuatorRF)
  Type 2 Element RF/1(Nodes) -> Nodes/1
  Type 2 Element RF/2(RF) -> RF/1
  Displ_cmd/1 -> Type 2 Element RF/3(Displacement)
  Constant/1 -> Type 2 Element RF/2(NumFreeDOF)
  Constant1/1 -> Type 2 Element RF/5(simulation)

== system RealtimeModel/Generate Element  Restoring Forces/Generate Type 3  Element Restoring Force Element 1 ==
  Displ_cmd : Inport  OutDataType=sfix(16)  OutScaling=2^0
  Constant : Constant  Value=Structure.NumFreeDOF  OutDataType=sfix(16)  OutScaling=2^0
  "Type 3 Element " : Subsystem  mask(Element Type 3){id=id}
      mask prompts: id "Element ID:"
      mask help: Enter the ID for this element corresponding with the input configuration file
  Type 3 Element RF : Stateflow chart  TreatAsAtomicUnit=on  SystemSampleTime=SampleRate
  Nodes : Outport  OutDataType=sfix(16)  OutScaling=2^0
  RF : Outport  Port=2  OutDataType=sfix(16)  OutScaling=2^0
  wires:
  "Type 3 Element "/5(bmy) -> Type 3 Element RF/5(bmy_init)
  "Type 3 Element "/4(pmx) -> Type 3 Element RF/4(pmx)
  "Type 3 Element "/3(a2) -> Type 3 Element RF/3(a2)
  "Type 3 Element "/2(a1) -> Type 3 Element RF/2(a1)
  Type 3 Element RF/1(Nodes) -> Nodes/1
  Type 3 Element RF/2(RF) -> RF/1
  "Type 3 Element "/1(Element) -> Type 3 Element RF/1(Element)
  Displ_cmd/1 -> Type 3 Element RF/7(Displacement)
  Constant/1 -> Type 3 Element RF/6(NumFreeDOF)

== system RealtimeModel/Generate Element  Restoring Forces/Generate Type 3  Element Restoring Force Element 10 ==
  Displ_cmd : Inport  OutDataType=sfix(16)  OutScaling=2^0
  Constant : Constant  Value=Structure.NumFreeDOF  OutDataType=sfix(16)  OutScaling=2^0
  "Type 3 Element " : Subsystem  mask(Element Type 3){id=id}
      mask prompts: id "Element ID:"
      mask help: Enter the ID for this element corresponding with the input configuration file
  Type 3 Element RF : Stateflow chart  TreatAsAtomicUnit=on  SystemSampleTime=SampleRate
  Nodes : Outport  OutDataType=sfix(16)  OutScaling=2^0
  RF : Outport  Port=2  OutDataType=sfix(16)  OutScaling=2^0
  wires:
  Constant/1 -> Type 3 Element RF/6(NumFreeDOF)
  Displ_cmd/1 -> Type 3 Element RF/7(Displacement)
  "Type 3 Element "/1(Element) -> Type 3 Element RF/1(Element)
  Type 3 Element RF/2(RF) -> RF/1
  Type 3 Element RF/1(Nodes) -> Nodes/1
  "Type 3 Element "/2(a1) -> Type 3 Element RF/2(a1)
  "Type 3 Element "/3(a2) -> Type 3 Element RF/3(a2)
  "Type 3 Element "/4(pmx) -> Type 3 Element RF/4(pmx)
  "Type 3 Element "/5(bmy) -> Type 3 Element RF/5(bmy_init)

== system RealtimeModel/Generate Element  Restoring Forces/Generate Type 3  Element Restoring Force Element 13 ==
  Displ_cmd : Inport  OutDataType=sfix(16)  OutScaling=2^0
  Constant : Constant  Value=Structure.NumFreeDOF  OutDataType=sfix(16)  OutScaling=2^0
  "Type 3 Element " : Subsystem  mask(Element Type 3){id=id}
      mask prompts: id "Element ID:"
      mask help: Enter the ID for this element corresponding with the input configuration file
  Type 3 Element RF : Stateflow chart  TreatAsAtomicUnit=on  SystemSampleTime=SampleRate
  Nodes : Outport  OutDataType=sfix(16)  OutScaling=2^0
  RF : Outport  Port=2  OutDataType=sfix(16)  OutScaling=2^0
  wires:
  Constant/1 -> Type 3 Element RF/6(NumFreeDOF)
  Displ_cmd/1 -> Type 3 Element RF/7(Displacement)
  "Type 3 Element "/1(Element) -> Type 3 Element RF/1(Element)
  Type 3 Element RF/2(RF) -> RF/1
  Type 3 Element RF/1(Nodes) -> Nodes/1
  "Type 3 Element "/2(a1) -> Type 3 Element RF/2(a1)
  "Type 3 Element "/3(a2) -> Type 3 Element RF/3(a2)
  "Type 3 Element "/4(pmx) -> Type 3 Element RF/4(pmx)
  "Type 3 Element "/5(bmy) -> Type 3 Element RF/5(bmy_init)

== system RealtimeModel/Generate Element  Restoring Forces/Generate Type 3  Element Restoring Force Element 16 ==
  Displ_cmd : Inport  OutDataType=sfix(16)  OutScaling=2^0
  Constant : Constant  Value=Structure.NumFreeDOF  OutDataType=sfix(16)  OutScaling=2^0
  "Type 3 Element " : Subsystem  mask(Element Type 3){id=id}
      mask prompts: id "Element ID:"
      mask help: Enter the ID for this element corresponding with the input configuration file
  Type 3 Element RF : Stateflow chart  TreatAsAtomicUnit=on  SystemSampleTime=SampleRate
  Nodes : Outport  OutDataType=sfix(16)  OutScaling=2^0
  RF : Outport  Port=2  OutDataType=sfix(16)  OutScaling=2^0
  wires:
  Constant/1 -> Type 3 Element RF/6(NumFreeDOF)
  Displ_cmd/1 -> Type 3 Element RF/7(Displacement)
  "Type 3 Element "/1(Element) -> Type 3 Element RF/1(Element)
  Type 3 Element RF/2(RF) -> RF/1
  Type 3 Element RF/1(Nodes) -> Nodes/1
  "Type 3 Element "/2(a1) -> Type 3 Element RF/2(a1)
  "Type 3 Element "/3(a2) -> Type 3 Element RF/3(a2)
  "Type 3 Element "/4(pmx) -> Type 3 Element RF/4(pmx)
  "Type 3 Element "/5(bmy) -> Type 3 Element RF/5(bmy_init)

== system RealtimeModel/Generate Element  Restoring Forces/Generate Type 3  Element Restoring Force Element 17 ==
  Displ_cmd : Inport  OutDataType=sfix(16)  OutScaling=2^0
  Constant : Constant  Value=Structure.NumFreeDOF  OutDataType=sfix(16)  OutScaling=2^0
  "Type 3 Element " : Subsystem  mask(Element Type 3){id=id}
      mask prompts: id "Element ID:"
      mask help: Enter the ID for this element corresponding with the input configuration file
  Type 3 Element RF : Stateflow chart  TreatAsAtomicUnit=on  SystemSampleTime=SampleRate
  Nodes : Outport  OutDataType=sfix(16)  OutScaling=2^0
  RF : Outport  Port=2  OutDataType=sfix(16)  OutScaling=2^0
  wires:
  "Type 3 Element "/5(bmy) -> Type 3 Element RF/5(bmy_init)
  "Type 3 Element "/4(pmx) -> Type 3 Element RF/4(pmx)
  "Type 3 Element "/3(a2) -> Type 3 Element RF/3(a2)
  "Type 3 Element "/2(a1) -> Type 3 Element RF/2(a1)
  Type 3 Element RF/1(Nodes) -> Nodes/1
  Type 3 Element RF/2(RF) -> RF/1
  "Type 3 Element "/1(Element) -> Type 3 Element RF/1(Element)
  Displ_cmd/1 -> Type 3 Element RF/7(Displacement)
  Constant/1 -> Type 3 Element RF/6(NumFreeDOF)

== system RealtimeModel/Generate Element  Restoring Forces/Generate Type 3  Element Restoring Force Element 18 ==
  Displ_cmd : Inport  OutDataType=sfix(16)  OutScaling=2^0
  Constant : Constant  Value=Structure.NumFreeDOF  OutDataType=sfix(16)  OutScaling=2^0
  "Type 3 Element " : Subsystem  mask(Element Type 3){id=id}
      mask prompts: id "Element ID:"
      mask help: Enter the ID for this element corresponding with the input configuration file
  Type 3 Element RF : Stateflow chart  TreatAsAtomicUnit=on  SystemSampleTime=SampleRate
  Nodes : Outport  OutDataType=sfix(16)  OutScaling=2^0
  RF : Outport  Port=2  OutDataType=sfix(16)  OutScaling=2^0
  wires:
  Constant/1 -> Type 3 Element RF/6(NumFreeDOF)
  Displ_cmd/1 -> Type 3 Element RF/7(Displacement)
  "Type 3 Element "/1(Element) -> Type 3 Element RF/1(Element)
  Type 3 Element RF/2(RF) -> RF/1
  Type 3 Element RF/1(Nodes) -> Nodes/1
  "Type 3 Element "/2(a1) -> Type 3 Element RF/2(a1)
  "Type 3 Element "/3(a2) -> Type 3 Element RF/3(a2)
  "Type 3 Element "/4(pmx) -> Type 3 Element RF/4(pmx)
  "Type 3 Element "/5(bmy) -> Type 3 Element RF/5(bmy_init)

== system RealtimeModel/Generate Element  Restoring Forces/Generate Type 3  Element Restoring Force Element 19 ==
  Displ_cmd : Inport  OutDataType=sfix(16)  OutScaling=2^0
  Constant : Constant  Value=Structure.NumFreeDOF  OutDataType=sfix(16)  OutScaling=2^0
  "Type 3 Element " : Subsystem  mask(Element Type 3){id=id}
      mask prompts: id "Element ID:"
      mask help: Enter the ID for this element corresponding with the input configuration file
  Type 3 Element RF : Stateflow chart  TreatAsAtomicUnit=on  SystemSampleTime=SampleRate
  Nodes : Outport  OutDataType=sfix(16)  OutScaling=2^0
  RF : Outport  Port=2  OutDataType=sfix(16)  OutScaling=2^0
  wires:
  "Type 3 Element "/5(bmy) -> Type 3 Element RF/5(bmy_init)
  "Type 3 Element "/4(pmx) -> Type 3 Element RF/4(pmx)
  "Type 3 Element "/3(a2) -> Type 3 Element RF/3(a2)
  "Type 3 Element "/2(a1) -> Type 3 Element RF/2(a1)
  Type 3 Element RF/1(Nodes) -> Nodes/1
  Type 3 Element RF/2(RF) -> RF/1
  "Type 3 Element "/1(Element) -> Type 3 Element RF/1(Element)
  Displ_cmd/1 -> Type 3 Element RF/7(Displacement)
  Constant/1 -> Type 3 Element RF/6(NumFreeDOF)
